simulink model "maglev"  (R2022a)
settings: Solver=VariableStepAuto  StartTime=0.0  StopTime=10.0  FixedStep=5e-10  RelTol=1e-3
settings Model: Creator=user  LastModifiedBy=user

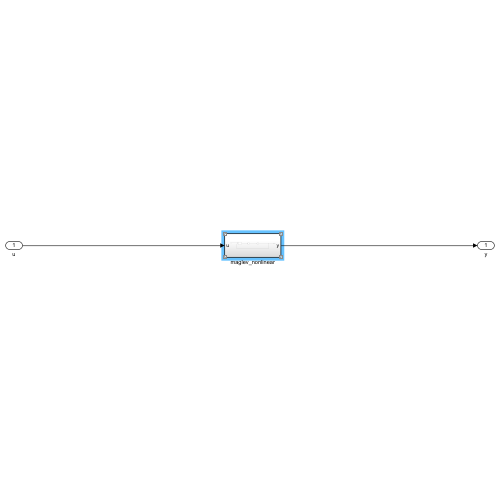
[thumbnail: Simulink's stored preview of the top-level diagram]
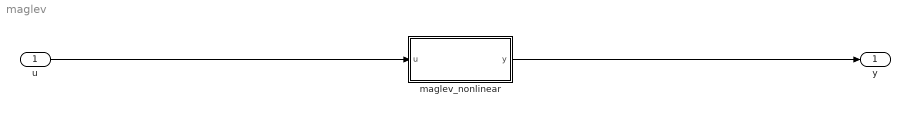
== system maglev ==
  u : Inport
  maglev_nonlinear : Subsystem
  y : Outport
  wires:
  u/1 -> maglev_nonlinear/1(u)
  maglev_nonlinear/1(y) -> y/1

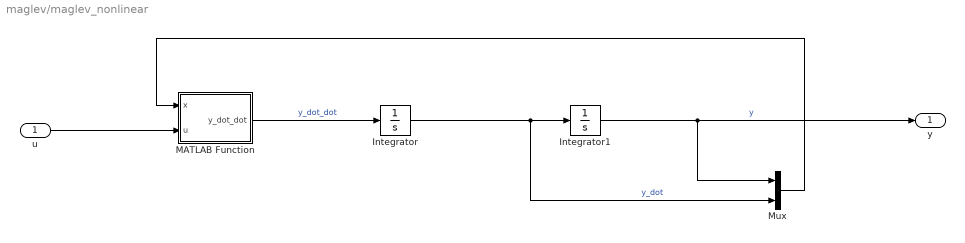
== system maglev/maglev_nonlinear ==
  u : Inport
  Integrator : Integrator
  Integrator1 : Integrator
  MATLAB Function : MATLAB Function  TreatAsAtomicUnit=on
  Mux : Mux  Inputs=2
  y : Outport
  wires:
  MATLAB Function/1(y_dot_dot) -> Integrator/1  "y_dot_dot"
  Integrator/1 -> Mux/2, Integrator1/1  "y_dot"
  Mux/1 -> MATLAB Function/1(x)
  Integrator1/1 -> Mux/1, y/1  "y"
  u/1 -> MATLAB Function/2(u)

== matlab function maglev/maglev_nonlinear/MATLAB Function ==
  data: x input; y_dot_dot output; u input
function y_dot_dot = fcn(x, u)

y_dot_dot = 9.8 - (u^2/x(1)^2);
